simulink model "V_1_2_SystemsmModelling_Control_Heat"  (R2020a)
settings: Solver=ode23t  StartTime=0.0  StopTime=10  MaxStep=2000.0  RelTol=1e-3
values from neighbouring files (symbols this model uses):
  InitialTemp = 300    [Setup.m]
undefined symbols (not defined in the file or in its folder): commanded_mass_flow, compressor_time_constant, condenser_length, copper_density, environment_temperature, evaporator_length, ground_temperature, max_throat_area, max_throat_temperature, min_throat_area, min_throat_temperature, pipe_diameter, pipe_thickness, target_temperature, temperature_delta, u_sat
libraries: fl_lib x46, refrigeration_lib x19, nesl_utility x9, fl_ps_legacy_lib x5
(part 2 of 2)

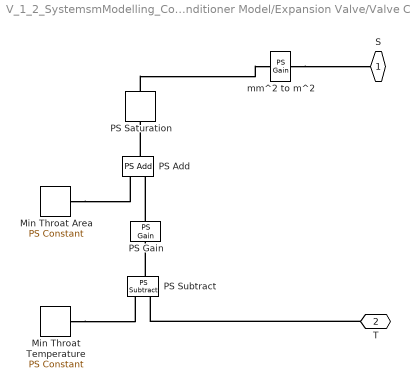
== system V_1_2_SystemsmModelling_Control_Heat/Air Conditioner Model/Expansion Valve/Valve Control ==
  Min Throat Area : fl_lib/Physical Signals/Sources/PS Constant  constant=min_throat_area
  Min Throat Temperature : fl_lib/Physical Signals/Sources/PS Constant  constant=min_throat_temperature
  PS Add : fl_ps_legacy_lib/Legacy Physical Signals/Functions/PS Add
      settings: SourceProductBaseCode=SS  InternalSimscapePortConfiguration="{\"Bottom\":[],\"Left\":[{\"id\":\"I1\",\"label\":\"\",\"type\":\"input\"},{\"id\":\"I2\",\"label\":\"\",\"type\":\"input\"}],\"Right\":[{\"id\":\"O\",\"label\":\"\",\"type\":\"output\"}],\"Top\":[]}"
  PS Gain : fl_ps_legacy_lib/Legacy Physical Signals/Functions/PS Gain  gain=(max_throat_area - min_throat_area)/(max_throat_temperature - min_throat_temperature)
  PS Saturation : fl_ps_legacy_lib/Legacy Physical Signals/Nonlinear Operators/PS Saturation  upper_limit=max_throat_area  lower_limit=min_throat_area
      settings: SourceProductBaseCode=SS  InternalSimscapePortConfiguration="{\"Bottom\":[],\"Left\":[{\"id\":\"I\",\"label\":\"\",\"type\":\"input\"}],\"Right\":[{\"id\":\"O\",\"label\":\"\",\"type\":\"output\"}],\"Top\":[]}"
  PS Subtract : fl_ps_legacy_lib/Legacy Physical Signals/Functions/PS Subtract
      settings: SourceProductBaseCode=SS
  mm^2 to m^2 : fl_ps_legacy_lib/Legacy Physical Signals/Functions/PS Gain  gain=1e-6
  S : PMIOPort  Side=Left
  T : PMIOPort  Port=2  Side=Right
  connections:
  mm^2 to m^2/RConn1 -- S/RConn1
  PS Saturation/RConn1 -- mm^2 to m^2/LConn1
  PS Subtract/RConn1 -- PS Gain/LConn1
  T/RConn1 -- PS Subtract/LConn1
  PS Add/RConn1 -- PS Saturation/LConn1
  Min Throat Area/RConn1 -- PS Add/LConn1
  Min Throat Temperature/RConn1 -- PS Subtract/LConn2
  PS Gain/RConn1 -- PS Add/LConn2

== system V_1_2_SystemsmModelling_Control_Heat/Air Conditioner Model/Refrigerator Compartment/Environment Temperature ==
  Constant : Constant  Value=environment_temperature
  Ideal Temperature Source : fl_lib/Thermal/Thermal Sources/Controlled Temperature Source
  Simulink-PS Converter : nesl_utility/Simulink-PS Converter  PhysicalDomain=network_engine_domain  SubClassName=ps_input  LeftPortType=input  RightPortType=output  PseudoPeriodic=off  Frequencies=[]  NoiseDistribution=none  NoiseParameters=[]  Unit=K  AffineConversion=off  FilteringAndDerivatives=zero  SimscapeFilterOrder=1  InputFilterTimeConstant=0.001  UdotUserProvided=1
  Thermal Reference : fl_lib/Thermal/Thermal Elements/Thermal Reference
  T : PMIOPort  Side=Left
  wires:
  Constant/1 -> Simulink-PS Converter/1
  connections:
  Ideal Temperature Source/RConn2 -- Thermal Reference/LConn1
  Ideal Temperature Source/RConn1 -- Simulink-PS Converter/RConn1
  Ideal Temperature Source/LConn1 -- T/RConn1

== system V_1_2_SystemsmModelling_Control_Heat/Air Conditioner Model/Refrigerator Compartment/Heat Flow Sensor ==
  Ideal Heat Flow Sensor : fl_lib/Thermal/Thermal Sensors/Heat Flow Rate Sensor
      settings: SourceProductBaseCode=SS
  B : PMIOPort  Side=Right
  A : PMIOPort  Port=2  Side=Left
  connections:
  Ideal Heat Flow Sensor/RConn2 -- B/RConn1
  Ideal Heat Flow Sensor/LConn1 -- A/RConn1

== system V_1_2_SystemsmModelling_Control_Heat/Air Conditioner Model/Refrigerator Compartment/Temperature Sensor ==
  Ideal Temperature Sensor : fl_lib/Thermal/Thermal Sensors/Temperature Sensor
  PS-Simulink Converter : nesl_utility/PS-Simulink Converter  PhysicalDomain=network_engine_domain  SubClassName=ps_output  LeftPortType=input  RightPortType=output  PseudoPeriodic=off  Frequencies=[]  Unit=K  AffineConversion=off
  Thermal Reference : fl_lib/Thermal/Thermal Elements/Thermal Reference
  A : PMIOPort  Side=Left
  T : Outport
  wires:
  PS-Simulink Converter/1 -> T/1
  connections:
  Ideal Temperature Sensor/LConn1 -- A/RConn1
  Thermal Reference/LConn1 -- Ideal Temperature Sensor/RConn1
  PS-Simulink Converter/LConn1 -- Ideal Temperature Sensor/RConn2
